simulink library "TetherTestLib"  (R2016a)
settings: Solver=ode45  StartTime=0.0  StopTime=10.0  RelTol=1e-3
libraries: TetherTestLib x1
settings Model: Creator=cjt79  LastModifiedBy=cjt79
settings DataIOCC: LimitDataPoints=on
settings DebuggingCC: AllowSymbolicDim=off

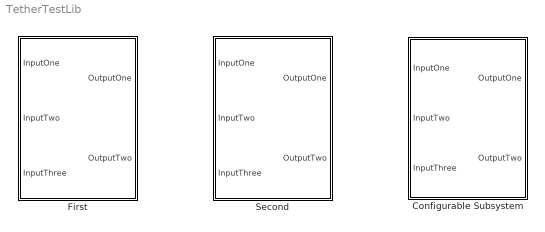
== system TetherTestLib ==
  Configurable Subsystem : Subsystem  BlockChoice=First
      settings: TemplateBlock=self  MemberBlocks=First,Second
  First : Subsystem
  Second : Subsystem

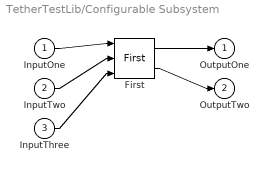
== system TetherTestLib/Configurable Subsystem ==
  InputOne : Inport
  InputTwo : Inport  Port=2
  InputThree : Inport  Port=3
  First : TetherTestLib/First
  OutputOne : Outport
  OutputTwo : Outport  Port=2
  wires:
  InputOne/1 -> First/1
  InputTwo/1 -> First/2
  InputThree/1 -> First/3
  First/1 -> OutputOne/1
  First/2 -> OutputTwo/1

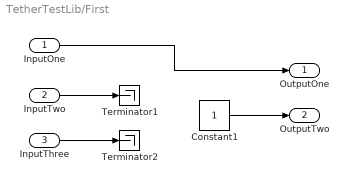
== system TetherTestLib/First ==
  InputOne : Inport
  InputTwo : Inport  Port=2
  InputThree : Inport  Port=3
  Constant1 : Constant
  Terminator1 : Terminator
  Terminator2 : Terminator
  OutputOne : Outport
  OutputTwo : Outport  Port=2
  wires:
  InputThree/1 -> Terminator2/1
  InputTwo/1 -> Terminator1/1
  InputOne/1 -> OutputOne/1
  Constant1/1 -> OutputTwo/1

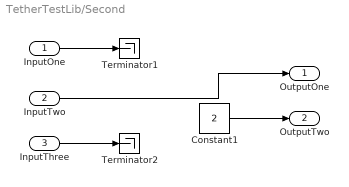
== system TetherTestLib/Second ==
  InputOne : Inport
  InputTwo : Inport  Port=2
  InputThree : Inport  Port=3
  Constant1 : Constant  Value=2
  Terminator1 : Terminator
  Terminator2 : Terminator
  OutputOne : Outport
  OutputTwo : Outport  Port=2
  wires:
  InputThree/1 -> Terminator2/1
  Constant1/1 -> OutputTwo/1
  InputOne/1 -> Terminator1/1
  InputTwo/1 -> OutputOne/1
